simulink model "Roll_Simulation"  (R2022b)
settings: Solver=VariableStepAuto  StartTime=0.0  StopTime=5  RelTol=1e-3
values from neighbouring files (symbols this model uses):
  N_RollRate_val = 20    [Roll_TF_Analysis.m]
  Ts_val = 0.01    [Roll_Root_Locus_Analysis.m]    (also in Roll_TF_Analysis.m)
settings Model: Creator=marcv  LastModifiedBy=marcv

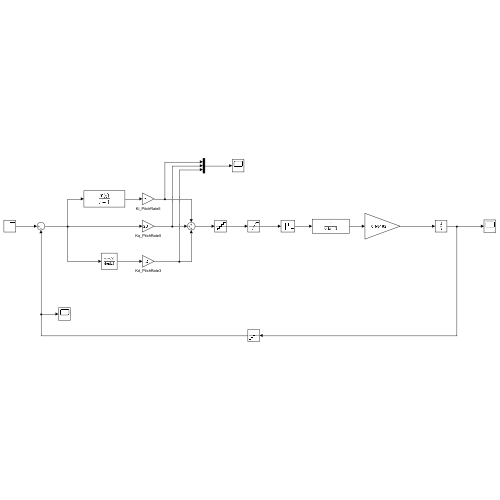
[thumbnail: Simulink's stored preview of the top-level diagram]
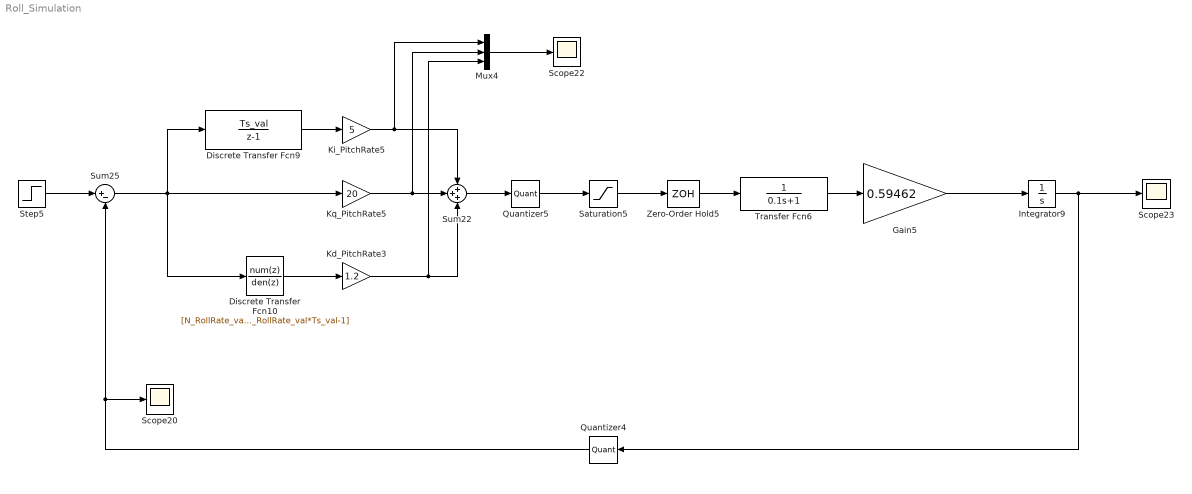
== system Roll_Simulation ==
  Discrete Transfer Fcn10 : DiscreteTransferFcn  Numerator=[N_RollRate_val, -N_RollRate_val]  Denominator=[1, N_RollRate_val*Ts_val-1]  SampleTime=Ts_val
  Discrete Transfer Fcn9 : DiscreteTransferFcn  Numerator=Ts_val  Denominator=[1,-1]  SampleTime=Ts_val
  Gain5 : Gain  Gain=0.59462
  Integrator9 : Integrator
  Kd_PitchRate3 : Gain  Gain=1.2
  Ki_PitchRate5 : Gain  Gain=5
  Kq_PitchRate5 : Gain  Gain=20
  Mux4 : Mux  Inputs=3
  Quantizer4 : Quantizer  QuantizationInterval=0.001
  Quantizer5 : Quantizer  QuantizationInterval=1
  Saturation5 : Saturate  UpperLimit=200  LowerLimit=-200
  Scope20 : Scope
  Scope22 : Scope
  Scope23 : Scope
  Step5 : Step  SampleTime=0
  Sum22 : Sum  Inputs=+++
  Sum25 : Sum  Inputs=|+-
  Transfer Fcn6 : TransferFcn  Denominator=[0.1 1]
  Zero-Order Hold5 : ZeroOrderHold  SampleTime=Ts_val
  wires:
  Integrator9/1 -> Quantizer4/1, Scope23/1
  Sum25/1 -> Discrete Transfer Fcn10/1, Kq_PitchRate5/1, Discrete Transfer Fcn9/1
  Gain5/1 -> Integrator9/1
  Mux4/1 -> Scope22/1
  Discrete Transfer Fcn10/1 -> Kd_PitchRate3/1
  Discrete Transfer Fcn9/1 -> Ki_PitchRate5/1
  Step5/1 -> Sum25/1
  Transfer Fcn6/1 -> Gain5/1
  Ki_PitchRate5/1 -> Sum22/1, Mux4/1
  Kq_PitchRate5/1 -> Mux4/2, Sum22/2
  Kd_PitchRate3/1 -> Mux4/3, Sum22/3
  Saturation5/1 -> Zero-Order Hold5/1
  Sum22/1 -> Quantizer5/1
  Quantizer5/1 -> Saturation5/1
  Zero-Order Hold5/1 -> Transfer Fcn6/1
  Quantizer4/1 -> Sum25/2, Scope20/1
